simulink model "snap2_f_200msps_64i_4096c"  (R2019a)
settings: Solver=VariableStepDiscrete  StartTime=0.0  StopTime=10.0  RelTol=1e-3
undefined symbols (not defined in the file or in its folder): datetime, posixtime
libraries: xbsIndex_r4 x21354, casper_library_misc x297, casper_library_delays x19, xps_library x14, casper_library_sources x4
(part 151 of 217)

== system snap2_f_200msps_64i_4096c/cosmic_ray/buffer_and_packetizer/transpose/bus_create4 ==
  in1 : Inport
  in2 : Inport  Port=2
  concatenate : xbsIndex_r4/Concat  num_inputs=2  dbl_ovrd=off  block_type=concat
  reinterpret1 : xbsIndex_r4/Reinterpret  force_arith_type=on  arith_type=Unsigned  force_bin_pt=on  bin_pt=0  block_type=reinterpret
      settings: infoedit="Changes signal type without altering the binary representation.   You can changed the signal between signed and unsigned, and relocate the binary point.<br><br>Hardware notes: In hardware this block costs nothing.<br><br>Example:  Suppose the input is 6 bits wide, signed, with 2 fractional bits, and the output is forced to unsigned with 0 fractional bits.  Then an input of -2.0 (1110.00 in binary 2's complement) becomes an output of 56 (111000 in binary)."
  reinterpret2 : xbsIndex_r4/Reinterpret  force_arith_type=on  arith_type=Unsigned  force_bin_pt=on  bin_pt=0  block_type=reinterpret
      settings: infoedit="Changes signal type without altering the binary representation.   You can changed the signal between signed and unsigned, and relocate the binary point.<br><br>Hardware notes: In hardware this block costs nothing.<br><br>Example:  Suppose the input is 6 bits wide, signed, with 2 fractional bits, and the output is forced to unsigned with 0 fractional bits.  Then an input of -2.0 (1110.00 in binary 2's complement) becomes an output of 56 (111000 in binary)."
  bus_out : Outport
  wires:
  concatenate/1 -> bus_out/1
  in1/1 -> reinterpret1/1
  reinterpret1/1 -> concatenate/1
  in2/1 -> reinterpret2/1
  reinterpret2/1 -> concatenate/2

== system snap2_f_200msps_64i_4096c/cosmic_ray/buffer_and_packetizer/transpose/bus_create5 ==
  in1 : Inport
  in2 : Inport  Port=2
  concatenate : xbsIndex_r4/Concat  num_inputs=2  dbl_ovrd=off  block_type=concat
  reinterpret1 : xbsIndex_r4/Reinterpret  force_arith_type=on  arith_type=Unsigned  force_bin_pt=on  bin_pt=0  block_type=reinterpret
      settings: infoedit="Changes signal type without altering the binary representation.   You can changed the signal between signed and unsigned, and relocate the binary point.<br><br>Hardware notes: In hardware this block costs nothing.<br><br>Example:  Suppose the input is 6 bits wide, signed, with 2 fractional bits, and the output is forced to unsigned with 0 fractional bits.  Then an input of -2.0 (1110.00 in binary 2's complement) becomes an output of 56 (111000 in binary)."
  reinterpret2 : xbsIndex_r4/Reinterpret  force_arith_type=on  arith_type=Unsigned  force_bin_pt=on  bin_pt=0  block_type=reinterpret
      settings: infoedit="Changes signal type without altering the binary representation.   You can changed the signal between signed and unsigned, and relocate the binary point.<br><br>Hardware notes: In hardware this block costs nothing.<br><br>Example:  Suppose the input is 6 bits wide, signed, with 2 fractional bits, and the output is forced to unsigned with 0 fractional bits.  Then an input of -2.0 (1110.00 in binary 2's complement) becomes an output of 56 (111000 in binary)."
  bus_out : Outport
  wires:
  reinterpret2/1 -> concatenate/2
  in2/1 -> reinterpret2/1
  reinterpret1/1 -> concatenate/1
  in1/1 -> reinterpret1/1
  concatenate/1 -> bus_out/1

== system snap2_f_200msps_64i_4096c/cosmic_ray/buffer_and_packetizer/transpose/bus_create6 ==
  in1 : Inport
  in2 : Inport  Port=2
  concatenate : xbsIndex_r4/Concat  num_inputs=2  dbl_ovrd=off  block_type=concat
  reinterpret1 : xbsIndex_r4/Reinterpret  force_arith_type=on  arith_type=Unsigned  force_bin_pt=on  bin_pt=0  block_type=reinterpret
      settings: infoedit="Changes signal type without altering the binary representation.   You can changed the signal between signed and unsigned, and relocate the binary point.<br><br>Hardware notes: In hardware this block costs nothing.<br><br>Example:  Suppose the input is 6 bits wide, signed, with 2 fractional bits, and the output is forced to unsigned with 0 fractional bits.  Then an input of -2.0 (1110.00 in binary 2's complement) becomes an output of 56 (111000 in binary)."
  reinterpret2 : xbsIndex_r4/Reinterpret  force_arith_type=on  arith_type=Unsigned  force_bin_pt=on  bin_pt=0  block_type=reinterpret
      settings: infoedit="Changes signal type without altering the binary representation.   You can changed the signal between signed and unsigned, and relocate the binary point.<br><br>Hardware notes: In hardware this block costs nothing.<br><br>Example:  Suppose the input is 6 bits wide, signed, with 2 fractional bits, and the output is forced to unsigned with 0 fractional bits.  Then an input of -2.0 (1110.00 in binary 2's complement) becomes an output of 56 (111000 in binary)."
  bus_out : Outport
  wires:
  reinterpret2/1 -> concatenate/2
  in2/1 -> reinterpret2/1
  reinterpret1/1 -> concatenate/1
  in1/1 -> reinterpret1/1
  concatenate/1 -> bus_out/1

== system snap2_f_200msps_64i_4096c/cosmic_ray/buffer_and_packetizer/transpose/bus_create7 ==
  in1 : Inport
  in2 : Inport  Port=2
  concatenate : xbsIndex_r4/Concat  num_inputs=2  dbl_ovrd=off  block_type=concat
  reinterpret1 : xbsIndex_r4/Reinterpret  force_arith_type=on  arith_type=Unsigned  force_bin_pt=on  bin_pt=0  block_type=reinterpret
      settings: infoedit="Changes signal type without altering the binary representation.   You can changed the signal between signed and unsigned, and relocate the binary point.<br><br>Hardware notes: In hardware this block costs nothing.<br><br>Example:  Suppose the input is 6 bits wide, signed, with 2 fractional bits, and the output is forced to unsigned with 0 fractional bits.  Then an input of -2.0 (1110.00 in binary 2's complement) becomes an output of 56 (111000 in binary)."
  reinterpret2 : xbsIndex_r4/Reinterpret  force_arith_type=on  arith_type=Unsigned  force_bin_pt=on  bin_pt=0  block_type=reinterpret
      settings: infoedit="Changes signal type without altering the binary representation.   You can changed the signal between signed and unsigned, and relocate the binary point.<br><br>Hardware notes: In hardware this block costs nothing.<br><br>Example:  Suppose the input is 6 bits wide, signed, with 2 fractional bits, and the output is forced to unsigned with 0 fractional bits.  Then an input of -2.0 (1110.00 in binary 2's complement) becomes an output of 56 (111000 in binary)."
  bus_out : Outport
  wires:
  concatenate/1 -> bus_out/1
  in1/1 -> reinterpret1/1
  reinterpret1/1 -> concatenate/1
  in2/1 -> reinterpret2/1
  reinterpret2/1 -> concatenate/2

== system snap2_f_200msps_64i_4096c/cosmic_ray/buffer_and_packetizer/transpose/bus_create8 ==
  in1 : Inport
  in2 : Inport  Port=2
  concatenate : xbsIndex_r4/Concat  num_inputs=2  dbl_ovrd=off  block_type=concat
  reinterpret1 : xbsIndex_r4/Reinterpret  force_arith_type=on  arith_type=Unsigned  force_bin_pt=on  bin_pt=0  block_type=reinterpret
      settings: infoedit="Changes signal type without altering the binary representation.   You can changed the signal between signed and unsigned, and relocate the binary point.<br><br>Hardware notes: In hardware this block costs nothing.<br><br>Example:  Suppose the input is 6 bits wide, signed, with 2 fractional bits, and the output is forced to unsigned with 0 fractional bits.  Then an input of -2.0 (1110.00 in binary 2's complement) becomes an output of 56 (111000 in binary)."
  reinterpret2 : xbsIndex_r4/Reinterpret  force_arith_type=on  arith_type=Unsigned  force_bin_pt=on  bin_pt=0  block_type=reinterpret
      settings: infoedit="Changes signal type without altering the binary representation.   You can changed the signal between signed and unsigned, and relocate the binary point.<br><br>Hardware notes: In hardware this block costs nothing.<br><br>Example:  Suppose the input is 6 bits wide, signed, with 2 fractional bits, and the output is forced to unsigned with 0 fractional bits.  Then an input of -2.0 (1110.00 in binary 2's complement) becomes an output of 56 (111000 in binary)."
  bus_out : Outport
  wires:
  reinterpret2/1 -> concatenate/2
  in2/1 -> reinterpret2/1
  reinterpret1/1 -> concatenate/1
  in1/1 -> reinterpret1/1
  concatenate/1 -> bus_out/1

== system snap2_f_200msps_64i_4096c/cosmic_ray/buffer_and_packetizer/transpose/bus_expand2 ==
  bus_in : Inport
  reinterpret{1..16} (16 alike) : xbsIndex_r4/Reinterpret  force_arith_type=on  arith_type="Signed  (2's comp)"  force_bin_pt=on  bin_pt=0  block_type=reinterpret
  slice1 : xbsIndex_r4/Slice  nbits=10  boolean_output=off  mode=Upper Bit Location + Width  bit1=-150  base1=MSB of Input  bit0=0  base0=LSB of Input  dbl_ovrd=off  block_type=slice
  slice10 : xbsIndex_r4/Slice  nbits=10  boolean_output=off  mode=Upper Bit Location + Width  bit1=-60  base1=MSB of Input  bit0=0  base0=LSB of Input  dbl_ovrd=off  block_type=slice
  slice11 : xbsIndex_r4/Slice  nbits=10  boolean_output=off  mode=Upper Bit Location + Width  bit1=-50  base1=MSB of Input  bit0=0  base0=LSB of Input  dbl_ovrd=off  block_type=slice
  slice12 : xbsIndex_r4/Slice  nbits=10  boolean_output=off  mode=Upper Bit Location + Width  bit1=-40  base1=MSB of Input  bit0=0  base0=LSB of Input  dbl_ovrd=off  block_type=slice
  slice13 : xbsIndex_r4/Slice  nbits=10  boolean_output=off  mode=Upper Bit Location + Width  bit1=-30  base1=MSB of Input  bit0=0  base0=LSB of Input  dbl_ovrd=off  block_type=slice
  slice14 : xbsIndex_r4/Slice  nbits=10  boolean_output=off  mode=Upper Bit Location + Width  bit1=-20  base1=MSB of Input  bit0=0  base0=LSB of Input  dbl_ovrd=off  block_type=slice
  slice15 : xbsIndex_r4/Slice  nbits=10  boolean_output=off  mode=Upper Bit Location + Width  bit1=-10  base1=MSB of Input  bit0=0  base0=LSB of Input  dbl_ovrd=off  block_type=slice
  slice16 : xbsIndex_r4/Slice  nbits=10  boolean_output=off  mode=Upper Bit Location + Width  bit1=0  base1=MSB of Input  bit0=0  base0=LSB of Input  dbl_ovrd=off  block_type=slice
  slice2 : xbsIndex_r4/Slice  nbits=10  boolean_output=off  mode=Upper Bit Location + Width  bit1=-140  base1=MSB of Input  bit0=0  base0=LSB of Input  dbl_ovrd=off  block_type=slice
  slice3 : xbsIndex_r4/Slice  nbits=10  boolean_output=off  mode=Upper Bit Location + Width  bit1=-130  base1=MSB of Input  bit0=0  base0=LSB of Input  dbl_ovrd=off  block_type=slice
  slice4 : xbsIndex_r4/Slice  nbits=10  boolean_output=off  mode=Upper Bit Location + Width  bit1=-120  base1=MSB of Input  bit0=0  base0=LSB of Input  dbl_ovrd=off  block_type=slice
  slice5 : xbsIndex_r4/Slice  nbits=10  boolean_output=off  mode=Upper Bit Location + Width  bit1=-110  base1=MSB of Input  bit0=0  base0=LSB of Input  dbl_ovrd=off  block_type=slice
  slice6 : xbsIndex_r4/Slice  nbits=10  boolean_output=off  mode=Upper Bit Location + Width  bit1=-100  base1=MSB of Input  bit0=0  base0=LSB of Input  dbl_ovrd=off  block_type=slice
  slice7 : xbsIndex_r4/Slice  nbits=10  boolean_output=off  mode=Upper Bit Location + Width  bit1=-90  base1=MSB of Input  bit0=0  base0=LSB of Input  dbl_ovrd=off  block_type=slice
  slice8 : xbsIndex_r4/Slice  nbits=10  boolean_output=off  mode=Upper Bit Location + Width  bit1=-80  base1=MSB of Input  bit0=0  base0=LSB of Input  dbl_ovrd=off  block_type=slice
  slice9 : xbsIndex_r4/Slice  nbits=10  boolean_output=off  mode=Upper Bit Location + Width  bit1=-70  base1=MSB of Input  bit0=0  base0=LSB of Input  dbl_ovrd=off  block_type=slice
  msb_out16 : Outport
  out15 : Outport  Port=2
  out14 : Outport  Port=3
  out13 : Outport  Port=4
  out12 : Outport  Port=5
  out11 : Outport  Port=6
  out10 : Outport  Port=7
  out9 : Outport  Port=8
  out8 : Outport  Port=9
  out7 : Outport  Port=10
  out6 : Outport  Port=11
  out5 : Outport  Port=12
  out4 : Outport  Port=13
  out3 : Outport  Port=14
  out2 : Outport  Port=15
  lsb_out1 : Outport  Port=16
  wires:
  bus_in/1 -> slice16/1, slice15/1, slice14/1, slice13/1, slice12/1, slice11/1, slice10/1, slice9/1, slice8/1, slice7/1, slice6/1, slice5/1, slice4/1, slice3/1, slice2/1, slice1/1
  slice16/1 -> reinterpret16/1
  reinterpret16/1 -> msb_out16/1
  slice15/1 -> reinterpret15/1
  reinterpret15/1 -> out15/1
  slice14/1 -> reinterpret14/1
  reinterpret14/1 -> out14/1
  slice13/1 -> reinterpret13/1
  reinterpret13/1 -> out13/1
  slice12/1 -> reinterpret12/1
  reinterpret12/1 -> out12/1
  slice11/1 -> reinterpret11/1
  reinterpret11/1 -> out11/1
  slice10/1 -> reinterpret10/1
  reinterpret10/1 -> out10/1
  slice9/1 -> reinterpret9/1
  reinterpret9/1 -> out9/1
  slice8/1 -> reinterpret8/1
  reinterpret8/1 -> out8/1
  slice7/1 -> reinterpret7/1
  reinterpret7/1 -> out7/1
  slice6/1 -> reinterpret6/1
  reinterpret6/1 -> out6/1
  slice5/1 -> reinterpret5/1
  reinterpret5/1 -> out5/1
  slice4/1 -> reinterpret4/1
  reinterpret4/1 -> out4/1
  slice3/1 -> reinterpret3/1
  reinterpret3/1 -> out3/1
  slice2/1 -> reinterpret2/1
  reinterpret2/1 -> out2/1
  slice1/1 -> reinterpret1/1
  reinterpret1/1 -> lsb_out1/1

== system snap2_f_200msps_64i_4096c/cosmic_ray/buffer_and_packetizer/transpose/square_transposer ==
  sync : Inport
  in0 : Inport  Port=2
  in1 : Inport  Port=3
  in2 : Inport  Port=4
  in3 : Inport  Port=5
  in4 : Inport  Port=6
  in5 : Inport  Port=7
  in6 : Inport  Port=8
  in7 : Inport  Port=9
  barrel_switcher : Subsystem  AncestorBlock=casper_library_reorder/barrel_switcher  mask(barrel_switcher){n_inputs=3, async=off}
      mask prompts: n_inputs "Number of Inputs: (2^?)"; async "Asynchronous operation"
      mask help:
      | Shifts input to right by amount specified on sel,
      | wrapping around into higher order bits.
      mask init:
      | barrel_switcher_init(gcb,...
      |     'n_inputs', n_inputs, ...
      |     'async', async);
      mask Help: eval('xlWeb(''http://casper.berkeley.edu/wiki/Barrel_switcher'')')
  counter : xbsIndex_r4/Counter  cnt_type=Free Running  cnt_to=Inf  operation=Down  start_count=0  cnt_by_val=1  arith_type=Unsigned  n_bits=n_inputs  bin_pt=0  load_pin=off  rst=on  en=off  explicit_period=on  period=1  use_behavioral_HDL=off  implementation=Fabric  dbl_ovrd=off  block_type=counter
  db0 : Subsystem  AncestorBlock=casper_library_delays/delay_slr  mask(delay_slr){DelayLen=7, async=off}
      mask prompts: DelayLen "Delay by:"; async "asynchronous operation"
      mask help: A delay block that uses slices (SLR16s) for its storage.
      mask init:
      | delay_slr_init(gcb, ...
      |     'DelayLen', DelayLen, ...
      |     'async', async);
  db1 : Subsystem  AncestorBlock=casper_library_delays/delay_slr  mask(delay_slr){DelayLen=6, async=off}
      mask prompts: DelayLen "Delay by:"; async "asynchronous operation"
      mask help: A delay block that uses slices (SLR16s) for its storage.
      mask init:
      | delay_slr_init(gcb, ...
      |     'DelayLen', DelayLen, ...
      |     'async', async);
  db2 : Subsystem  AncestorBlock=casper_library_delays/delay_slr  mask(delay_slr){DelayLen=5, async=off}
      mask prompts: DelayLen "Delay by:"; async "asynchronous operation"
      mask help: A delay block that uses slices (SLR16s) for its storage.
      mask init:
      | delay_slr_init(gcb, ...
      |     'DelayLen', DelayLen, ...
      |     'async', async);
  db3 : Subsystem  AncestorBlock=casper_library_delays/delay_slr  mask(delay_slr){DelayLen=4, async=off}
      mask prompts: DelayLen "Delay by:"; async "asynchronous operation"
      mask help: A delay block that uses slices (SLR16s) for its storage.
      mask init:
      | delay_slr_init(gcb, ...
      |     'DelayLen', DelayLen, ...
      |     'async', async);
  db4 : Subsystem  AncestorBlock=casper_library_delays/delay_slr  mask(delay_slr){DelayLen=3, async=off}
      mask prompts: DelayLen "Delay by:"; async "asynchronous operation"
      mask help: A delay block that uses slices (SLR16s) for its storage.
      mask init:
      | delay_slr_init(gcb, ...
      |     'DelayLen', DelayLen, ...
      |     'async', async);
  db5 : Subsystem  AncestorBlock=casper_library_delays/delay_slr  mask(delay_slr){DelayLen=2, async=off}
      mask prompts: DelayLen "Delay by:"; async "asynchronous operation"
      mask help: A delay block that uses slices (SLR16s) for its storage.
      mask init:
      | delay_slr_init(gcb, ...
      |     'DelayLen', DelayLen, ...
      |     'async', async);
  db6 : Subsystem  AncestorBlock=casper_library_delays/delay_slr  mask(delay_slr){DelayLen=1, async=off}
      mask prompts: DelayLen "Delay by:"; async "asynchronous operation"
      mask help: A delay block that uses slices (SLR16s) for its storage.
      mask init:
      | delay_slr_init(gcb, ...
      |     'DelayLen', DelayLen, ...
      |     'async', async);
  df1 : Subsystem  AncestorBlock=casper_library_delays/delay_slr  mask(delay_slr){DelayLen=1, async=off}
      mask prompts: DelayLen "Delay by:"; async "asynchronous operation"
      mask help: A delay block that uses slices (SLR16s) for its storage.
      mask init:
      | delay_slr_init(gcb, ...
      |     'DelayLen', DelayLen, ...
      |     'async', async);
  df2 : Subsystem  AncestorBlock=casper_library_delays/delay_slr  mask(delay_slr){DelayLen=2, async=off}
      mask prompts: DelayLen "Delay by:"; async "asynchronous operation"
      mask help: A delay block that uses slices (SLR16s) for its storage.
      mask init:
      | delay_slr_init(gcb, ...
      |     'DelayLen', DelayLen, ...
      |     'async', async);
  df3 : Subsystem  AncestorBlock=casper_library_delays/delay_slr  mask(delay_slr){DelayLen=3, async=off}
      mask prompts: DelayLen "Delay by:"; async "asynchronous operation"
      mask help: A delay block that uses slices (SLR16s) for its storage.
      mask init:
      | delay_slr_init(gcb, ...
      |     'DelayLen', DelayLen, ...
      |     'async', async);
  df4 : Subsystem  AncestorBlock=casper_library_delays/delay_slr  mask(delay_slr){DelayLen=4, async=off}
      mask prompts: DelayLen "Delay by:"; async "asynchronous operation"
      mask help: A delay block that uses slices (SLR16s) for its storage.
      mask init:
      | delay_slr_init(gcb, ...
      |     'DelayLen', DelayLen, ...
      |     'async', async);
  df5 : Subsystem  AncestorBlock=casper_library_delays/delay_slr  mask(delay_slr){DelayLen=5, async=off}
      mask prompts: DelayLen "Delay by:"; async "asynchronous operation"
      mask help: A delay block that uses slices (SLR16s) for its storage.
      mask init:
      | delay_slr_init(gcb, ...
      |     'DelayLen', DelayLen, ...
      |     'async', async);
  df6 : Subsystem  AncestorBlock=casper_library_delays/delay_slr  mask(delay_slr){DelayLen=6, async=off}
      mask prompts: DelayLen "Delay by:"; async "asynchronous operation"
      mask help: A delay block that uses slices (SLR16s) for its storage.
      mask init:
      | delay_slr_init(gcb, ...
      |     'DelayLen', DelayLen, ...
      |     'async', async);
  df7 : Subsystem  AncestorBlock=casper_library_delays/delay_slr  mask(delay_slr){DelayLen=7, async=off}
      mask prompts: DelayLen "Delay by:"; async "asynchronous operation"
      mask help: A delay block that uses slices (SLR16s) for its storage.
      mask init:
      | delay_slr_init(gcb, ...
      |     'DelayLen', DelayLen, ...
      |     'async', async);
  dsync : Subsystem  AncestorBlock=casper_library_delays/delay_slr  mask(delay_slr){DelayLen=7, async=off}
      mask prompts: DelayLen "Delay by:"; async "asynchronous operation"
      mask help: A delay block that uses slices (SLR16s) for its storage.
      mask init:
      | delay_slr_init(gcb, ...
      |     'DelayLen', DelayLen, ...
      |     'async', async);
  sync_out : Outport
  out0 : Outport  Port=2
  out1 : Outport  Port=3
  out2 : Outport  Port=4
  out3 : Outport  Port=5
  out4 : Outport  Port=6
  out5 : Outport  Port=7
  out6 : Outport  Port=8
  out7 : Outport  Port=9
  wires:
  sync/1 -> counter/1, barrel_switcher/2(sync_in)
  dsync/1(dout) -> sync_out/1
  counter/1 -> barrel_switcher/1(sel)
  barrel_switcher/1(sync_out) -> dsync/1(din)
  in0/1 -> barrel_switcher/3(In1)
  barrel_switcher/2(Out1) -> db0/1(din)
  db0/1(dout) -> out0/1
  in1/1 -> df1/1(din)
  df1/1(dout) -> barrel_switcher/10(In8)
  barrel_switcher/3(Out2) -> db1/1(din)
  db1/1(dout) -> out1/1
  in2/1 -> df2/1(din)
  df2/1(dout) -> barrel_switcher/9(In7)
  barrel_switcher/4(Out3) -> db2/1(din)
  db2/1(dout) -> out2/1
  in3/1 -> df3/1(din)
  df3/1(dout) -> barrel_switcher/8(In6)
  barrel_switcher/5(Out4) -> db3/1(din)
  db3/1(dout) -> out3/1
  in4/1 -> df4/1(din)
  df4/1(dout) -> barrel_switcher/7(In5)
  barrel_switcher/6(Out5) -> db4/1(din)
  db4/1(dout) -> out4/1
  in5/1 -> df5/1(din)
  df5/1(dout) -> barrel_switcher/6(In4)
  barrel_switcher/7(Out6) -> db5/1(din)
  db5/1(dout) -> out5/1
  in6/1 -> df6/1(din)
  df6/1(dout) -> barrel_switcher/5(In3)
  barrel_switcher/8(Out7) -> db6/1(din)
  db6/1(dout) -> out6/1
  in7/1 -> df7/1(din)
  df7/1(dout) -> barrel_switcher/4(In2)
  barrel_switcher/9(Out8) -> out7/1

== system snap2_f_200msps_64i_4096c/cosmic_ray/coincidence_trigger/4pt_avg/bus_addsub ==
  a : Inport
  b : Inport  Port=2
  a_debus : Subsystem  AncestorBlock=casper_library_flow_control/bus_expand  mask(bus_expand){mode=divisions of arbitrary size, outputNum=1, outputWidth=[24  24  24  24  24  24  24  24  24  24  24  24  24  24  24  24  24  24  24  24  24  24  24  24  24  24  24  24  24  24  24  24  24  24  24  24  24  24  24  24  24  24  24  24  24  24  24  24  24  24  24  24  24  24  24  24  24  24  24  24  24  24  24  24], outputBinaryPt=[0  0  0  0  0  0  0  0  0  0  0  0  0  0  0  0  0  0  0  0  0  0  0  0  0  0  0  0  0  0  0  0  0  0  0  0  0  0  0  0  0  0  0  0  0  0  0  0  0  0  0  0  0  0  0  0  0  0  0  0  0  0  0  0], outputArithmeticType=[1  1  1  1  1  1  1  1  1  1  1  1  1  1  1  1  1  1  1  1  1  1  1  1  1  1  1  1  1  1  1  1  1  1  1  1  1  1  1  1  1  1  1  1  1  1  1  1  1  1  1  1  1  1  1  1  1  1  1  1  1  1  1  1], show_format=on, outputToWorkspace=off, variablePrefix=, outputToModelAsWell=on}
      mask prompts: outputNum "Number of outputs:"; outputWidth "Output width [msb ... lsb]:"; outputBinaryPt "Output binary point position [msb ... lsb]:"; outputArithmeticType "Output arithmetic type (ufix=0, fix=1, bool=2) [msb ... lsb]:"; show_format "Print format string?"; outputToWorkspace "Output to workspace?"; variablePrefix "Variable name prefix:"; outputToModelAsWell "Output to model as well?"
      mask help:
      | Expands a 'bus' made using a bus_create or Xilinx
      | concat block.
      | The input will be divided into the specified number
      | of outputs with the specified arithmetic types.
      | Divisions are made from most significant bit.
      mask init: same as snap2_f_200msps_64i_4096c/autocorr/bus_expand
      settings: AttributesFormatString=64 outputs: f24.0,f24.0,f24.0,f24.0,f24.0,f24.0,f24.0,f24.0,f24.0,f24.0,f24.0,f24.0,f24.0,f24.0,f24.0,f24.0,f24.0,f24.0,f24.0,f24.0,f24.0,f24.0,f24.0,f24.0,f24.0,f24.0,f24.0,f24.0,f24.0,f24.0,f24.0,f24.0,f24.0,f24.0,f24.0,f24.0,f24.0,f24.0,f24.0,f24.0,f24.0,f24.0,f24.0,f24.0,f24.0,f24.0,f24.0,f24.0,f24.0,f24.0,f24.0,f24.0,f24.0,f24.0,f24.0,f24.0,f24.0,f24.0,f24.0,f24.0,f24.0,f24.0,f24.0,f24.0,
      mask TypeOptions mode: divisions of equal size | divisions of arbitrary size
      mask Callback mode: bus_expand_callback();
      mask Callback outputWidth: bus_expand_callback();
      mask Callback outputToWorkspace: bus_expand_callback();
  addsub{1..64} (64 alike) : xbsIndex_r4/AddSub  mode=Addition  use_carryin=off  use_carryout=off  en=off  latency=1  precision=User Defined  arith_type="Signed  (2's comp)"  n_bits=25  bin_pt=0  quantization=Truncate  overflow=Wrap  use_behavioral_HDL=on  hw_selection=Fabric  pipelined=on  dbl_ovrd=off  block_type=addsub
  b_debus : Subsystem  AncestorBlock=casper_library_flow_control/bus_expand  mask(bus_expand){mode=divisions of arbitrary size, outputNum=1, outputWidth=[24  24  24  24  24  24  24  24  24  24  24  24  24  24  24  24  24  24  24  24  24  24  24  24  24  24  24  24  24  24  24  24  24  24  24  24  24  24  24  24  24  24  24  24  24  24  24  24  24  24  24  24  24  24  24  24  24  24  24  24  24  24  24  24], outputBinaryPt=[0  0  0  0  0  0  0  0  0  0  0  0  0  0  0  0  0  0  0  0  0  0  0  0  0  0  0  0  0  0  0  0  0  0  0  0  0  0  0  0  0  0  0  0  0  0  0  0  0  0  0  0  0  0  0  0  0  0  0  0  0  0  0  0], outputArithmeticType=[1  1  1  1  1  1  1  1  1  1  1  1  1  1  1  1  1  1  1  1  1  1  1  1  1  1  1  1  1  1  1  1  1  1  1  1  1  1  1  1  1  1  1  1  1  1  1  1  1  1  1  1  1  1  1  1  1  1  1  1  1  1  1  1], show_format=on, outputToWorkspace=off, variablePrefix=, outputToModelAsWell=on}
      mask prompts: outputNum "Number of outputs:"; outputWidth "Output width [msb ... lsb]:"; outputBinaryPt "Output binary point position [msb ... lsb]:"; outputArithmeticType "Output arithmetic type (ufix=0, fix=1, bool=2) [msb ... lsb]:"; show_format "Print format string?"; outputToWorkspace "Output to workspace?"; variablePrefix "Variable name prefix:"; outputToModelAsWell "Output to model as well?"
      mask help:
      | Expands a 'bus' made using a bus_create or Xilinx
      | concat block.
      | The input will be divided into the specified number
      | of outputs with the specified arithmetic types.
      | Divisions are made from most significant bit.
      mask init: same as snap2_f_200msps_64i_4096c/autocorr/bus_expand
      settings: AttributesFormatString=64 outputs: f24.0,f24.0,f24.0,f24.0,f24.0,f24.0,f24.0,f24.0,f24.0,f24.0,f24.0,f24.0,f24.0,f24.0,f24.0,f24.0,f24.0,f24.0,f24.0,f24.0,f24.0,f24.0,f24.0,f24.0,f24.0,f24.0,f24.0,f24.0,f24.0,f24.0,f24.0,f24.0,f24.0,f24.0,f24.0,f24.0,f24.0,f24.0,f24.0,f24.0,f24.0,f24.0,f24.0,f24.0,f24.0,f24.0,f24.0,f24.0,f24.0,f24.0,f24.0,f24.0,f24.0,f24.0,f24.0,f24.0,f24.0,f24.0,f24.0,f24.0,f24.0,f24.0,f24.0,f24.0,
      mask TypeOptions mode: divisions of equal size | divisions of arbitrary size
      mask Callback mode: bus_expand_callback();
      mask Callback outputWidth: bus_expand_callback();
      mask Callback outputToWorkspace: bus_expand_callback();
  op_bussify : Subsystem  AncestorBlock=casper_library_flow_control/bus_create  mask(bus_create){inputNum=64}
      mask prompts: inputNum "Number of inputs:"
      mask init:
      | bus_create_init(gcb,...
      |     'inputNum', inputNum);
  dout : Outport
  wires:
  a/1 -> a_debus/1(bus_in)
  b/1 -> b_debus/1(bus_in)
  a_debus/1(msb_out64) -> addsub1/1
  b_debus/1(msb_out64) -> addsub1/2
  a_debus/2(out63) -> addsub2/1
  b_debus/2(out63) -> addsub2/2
  a_debus/3(out62) -> addsub3/1
  b_debus/3(out62) -> addsub3/2
  a_debus/4(out61) -> addsub4/1
  b_debus/4(out61) -> addsub4/2
  a_debus/5(out60) -> addsub5/1
  b_debus/5(out60) -> addsub5/2
  a_debus/6(out59) -> addsub6/1
  b_debus/6(out59) -> addsub6/2
  a_debus/7(out58) -> addsub7/1
  b_debus/7(out58) -> addsub7/2
  a_debus/8(out57) -> addsub8/1
  b_debus/8(out57) -> addsub8/2
  a_debus/9(out56) -> addsub9/1
  b_debus/9(out56) -> addsub9/2
  a_debus/10(out55) -> addsub10/1
  b_debus/10(out55) -> addsub10/2
  a_debus/11(out54) -> addsub11/1
  b_debus/11(out54) -> addsub11/2
  a_debus/12(out53) -> addsub12/1
  b_debus/12(out53) -> addsub12/2
  a_debus/13(out52) -> addsub13/1
  b_debus/13(out52) -> addsub13/2
  a_debus/14(out51) -> addsub14/1
  b_debus/14(out51) -> addsub14/2
  a_debus/15(out50) -> addsub15/1
  b_debus/15(out50) -> addsub15/2
  a_debus/16(out49) -> addsub16/1
  b_debus/16(out49) -> addsub16/2
  a_debus/17(out48) -> addsub17/1
  b_debus/17(out48) -> addsub17/2
  a_debus/18(out47) -> addsub18/1
  b_debus/18(out47) -> addsub18/2
  a_debus/19(out46) -> addsub19/1
  b_debus/19(out46) -> addsub19/2
  a_debus/20(out45) -> addsub20/1
  b_debus/20(out45) -> addsub20/2
  a_debus/21(out44) -> addsub21/1
  b_debus/21(out44) -> addsub21/2
  a_debus/22(out43) -> addsub22/1
  b_debus/22(out43) -> addsub22/2
  a_debus/23(out42) -> addsub23/1
  b_debus/23(out42) -> addsub23/2
  a_debus/24(out41) -> addsub24/1
  b_debus/24(out41) -> addsub24/2
  a_debus/25(out40) -> addsub25/1
  b_debus/25(out40) -> addsub25/2
  a_debus/26(out39) -> addsub26/1
  b_debus/26(out39) -> addsub26/2
  a_debus/27(out38) -> addsub27/1
  b_debus/27(out38) -> addsub27/2
  a_debus/28(out37) -> addsub28/1
  b_debus/28(out37) -> addsub28/2
  a_debus/29(out36) -> addsub29/1
  b_debus/29(out36) -> addsub29/2
  a_debus/30(out35) -> addsub30/1
  b_debus/30(out35) -> addsub30/2
  a_debus/31(out34) -> addsub31/1
  b_debus/31(out34) -> addsub31/2
  a_debus/32(out33) -> addsub32/1
  b_debus/32(out33) -> addsub32/2
  a_debus/33(out32) -> addsub33/1
  b_debus/33(out32) -> addsub33/2
  a_debus/34(out31) -> addsub34/1
  b_debus/34(out31) -> addsub34/2
  a_debus/35(out30) -> addsub35/1
  b_debus/35(out30) -> addsub35/2
  a_debus/36(out29) -> addsub36/1
  b_debus/36(out29) -> addsub36/2
  a_debus/37(out28) -> addsub37/1
  b_debus/37(out28) -> addsub37/2
  a_debus/38(out27) -> addsub38/1
  b_debus/38(out27) -> addsub38/2
  a_debus/39(out26) -> addsub39/1
  b_debus/39(out26) -> addsub39/2
  a_debus/40(out25) -> addsub40/1
  b_debus/40(out25) -> addsub40/2
  a_debus/41(out24) -> addsub41/1
  b_debus/41(out24) -> addsub41/2
  a_debus/42(out23) -> addsub42/1
  b_debus/42(out23) -> addsub42/2
  a_debus/43(out22) -> addsub43/1
  b_debus/43(out22) -> addsub43/2
  a_debus/44(out21) -> addsub44/1
  b_debus/44(out21) -> addsub44/2
  a_debus/45(out20) -> addsub45/1
  b_debus/45(out20) -> addsub45/2
  a_debus/46(out19) -> addsub46/1
  b_debus/46(out19) -> addsub46/2
  a_debus/47(out18) -> addsub47/1
  b_debus/47(out18) -> addsub47/2
  a_debus/48(out17) -> addsub48/1
  b_debus/48(out17) -> addsub48/2
  a_debus/49(out16) -> addsub49/1
  b_debus/49(out16) -> addsub49/2
  a_debus/50(out15) -> addsub50/1
  b_debus/50(out15) -> addsub50/2
  a_debus/51(out14) -> addsub51/1
  b_debus/51(out14) -> addsub51/2
  a_debus/52(out13) -> addsub52/1
  b_debus/52(out13) -> addsub52/2
  a_debus/53(out12) -> addsub53/1
  b_debus/53(out12) -> addsub53/2
  a_debus/54(out11) -> addsub54/1
  b_debus/54(out11) -> addsub54/2
  a_debus/55(out10) -> addsub55/1
  b_debus/55(out10) -> addsub55/2
  a_debus/56(out9) -> addsub56/1
  b_debus/56(out9) -> addsub56/2
  a_debus/57(out8) -> addsub57/1
  b_debus/57(out8) -> addsub57/2
  a_debus/58(out7) -> addsub58/1
  b_debus/58(out7) -> addsub58/2
  a_debus/59(out6) -> addsub59/1
  b_debus/59(out6) -> addsub59/2
  a_debus/60(out5) -> addsub60/1
  b_debus/60(out5) -> addsub60/2
  a_debus/61(out4) -> addsub61/1
  b_debus/61(out4) -> addsub61/2
  a_debus/62(out3) -> addsub62/1
  b_debus/62(out3) -> addsub62/2
  a_debus/63(out2) -> addsub63/1
  b_debus/63(out2) -> addsub63/2
  a_debus/64(lsb_out1) -> addsub64/1
  b_debus/64(lsb_out1) -> addsub64/2
  addsub1/1 -> op_bussify/1(in1)
  addsub2/1 -> op_bussify/2(in2)
  addsub3/1 -> op_bussify/3(in3)
  addsub4/1 -> op_bussify/4(in4)
  addsub5/1 -> op_bussify/5(in5)
  addsub6/1 -> op_bussify/6(in6)
  addsub7/1 -> op_bussify/7(in7)
  addsub8/1 -> op_bussify/8(in8)
  addsub9/1 -> op_bussify/9(in9)
  addsub10/1 -> op_bussify/10(in10)
  addsub11/1 -> op_bussify/11(in11)
  addsub12/1 -> op_bussify/12(in12)
  addsub13/1 -> op_bussify/13(in13)
  addsub14/1 -> op_bussify/14(in14)
  addsub15/1 -> op_bussify/15(in15)
  addsub16/1 -> op_bussify/16(in16)
  addsub17/1 -> op_bussify/17(in17)
  addsub18/1 -> op_bussify/18(in18)
  addsub19/1 -> op_bussify/19(in19)
  addsub20/1 -> op_bussify/20(in20)
  addsub21/1 -> op_bussify/21(in21)
  addsub22/1 -> op_bussify/22(in22)
  addsub23/1 -> op_bussify/23(in23)
  addsub24/1 -> op_bussify/24(in24)
  addsub25/1 -> op_bussify/25(in25)
  addsub26/1 -> op_bussify/26(in26)
  addsub27/1 -> op_bussify/27(in27)
  addsub28/1 -> op_bussify/28(in28)
  addsub29/1 -> op_bussify/29(in29)
  addsub30/1 -> op_bussify/30(in30)
  addsub31/1 -> op_bussify/31(in31)
  addsub32/1 -> op_bussify/32(in32)
  addsub33/1 -> op_bussify/33(in33)
  addsub34/1 -> op_bussify/34(in34)
  addsub35/1 -> op_bussify/35(in35)
  addsub36/1 -> op_bussify/36(in36)
  addsub37/1 -> op_bussify/37(in37)
  addsub38/1 -> op_bussify/38(in38)
  addsub39/1 -> op_bussify/39(in39)
  addsub40/1 -> op_bussify/40(in40)
  addsub41/1 -> op_bussify/41(in41)
  addsub42/1 -> op_bussify/42(in42)
  addsub43/1 -> op_bussify/43(in43)
  addsub44/1 -> op_bussify/44(in44)
  addsub45/1 -> op_bussify/45(in45)
  addsub46/1 -> op_bussify/46(in46)
  addsub47/1 -> op_bussify/47(in47)
  addsub48/1 -> op_bussify/48(in48)
  addsub49/1 -> op_bussify/49(in49)
  addsub50/1 -> op_bussify/50(in50)
  addsub51/1 -> op_bussify/51(in51)
  addsub52/1 -> op_bussify/52(in52)
  addsub53/1 -> op_bussify/53(in53)
  addsub54/1 -> op_bussify/54(in54)
  addsub55/1 -> op_bussify/55(in55)
  addsub56/1 -> op_bussify/56(in56)
  addsub57/1 -> op_bussify/57(in57)
  addsub58/1 -> op_bussify/58(in58)
  addsub59/1 -> op_bussify/59(in59)
  addsub60/1 -> op_bussify/60(in60)
  addsub61/1 -> op_bussify/61(in61)
  addsub62/1 -> op_bussify/62(in62)
  addsub63/1 -> op_bussify/63(in63)
  addsub64/1 -> op_bussify/64(in64)
  op_bussify/1(bus_out) -> dout/1

== system snap2_f_200msps_64i_4096c/cosmic_ray/coincidence_trigger/4pt_avg/bus_addsub1 ==
  a : Inport
  b : Inport  Port=2
  a_debus : Subsystem  AncestorBlock=casper_library_flow_control/bus_expand  mask(bus_expand){mode=divisions of arbitrary size, outputNum=1, outputWidth=[24  24  24  24  24  24  24  24  24  24  24  24  24  24  24  24  24  24  24  24  24  24  24  24  24  24  24  24  24  24  24  24  24  24  24  24  24  24  24  24  24  24  24  24  24  24  24  24  24  24  24  24  24  24  24  24  24  24  24  24  24  24  24  24], outputBinaryPt=[0  0  0  0  0  0  0  0  0  0  0  0  0  0  0  0  0  0  0  0  0  0  0  0  0  0  0  0  0  0  0  0  0  0  0  0  0  0  0  0  0  0  0  0  0  0  0  0  0  0  0  0  0  0  0  0  0  0  0  0  0  0  0  0], outputArithmeticType=[1  1  1  1  1  1  1  1  1  1  1  1  1  1  1  1  1  1  1  1  1  1  1  1  1  1  1  1  1  1  1  1  1  1  1  1  1  1  1  1  1  1  1  1  1  1  1  1  1  1  1  1  1  1  1  1  1  1  1  1  1  1  1  1], show_format=on, outputToWorkspace=off, variablePrefix=, outputToModelAsWell=on}
      mask prompts: outputNum "Number of outputs:"; outputWidth "Output width [msb ... lsb]:"; outputBinaryPt "Output binary point position [msb ... lsb]:"; outputArithmeticType "Output arithmetic type (ufix=0, fix=1, bool=2) [msb ... lsb]:"; show_format "Print format string?"; outputToWorkspace "Output to workspace?"; variablePrefix "Variable name prefix:"; outputToModelAsWell "Output to model as well?"
      mask help:
      | Expands a 'bus' made using a bus_create or Xilinx
      | concat block.
      | The input will be divided into the specified number
      | of outputs with the specified arithmetic types.
      | Divisions are made from most significant bit.
      mask init: same as snap2_f_200msps_64i_4096c/autocorr/bus_expand
      settings: AttributesFormatString=64 outputs: f24.0,f24.0,f24.0,f24.0,f24.0,f24.0,f24.0,f24.0,f24.0,f24.0,f24.0,f24.0,f24.0,f24.0,f24.0,f24.0,f24.0,f24.0,f24.0,f24.0,f24.0,f24.0,f24.0,f24.0,f24.0,f24.0,f24.0,f24.0,f24.0,f24.0,f24.0,f24.0,f24.0,f24.0,f24.0,f24.0,f24.0,f24.0,f24.0,f24.0,f24.0,f24.0,f24.0,f24.0,f24.0,f24.0,f24.0,f24.0,f24.0,f24.0,f24.0,f24.0,f24.0,f24.0,f24.0,f24.0,f24.0,f24.0,f24.0,f24.0,f24.0,f24.0,f24.0,f24.0,
      mask TypeOptions mode: divisions of equal size | divisions of arbitrary size
      mask Callback mode: bus_expand_callback();
      mask Callback outputWidth: bus_expand_callback();
      mask Callback outputToWorkspace: bus_expand_callback();
  addsub{1..64} (64 alike) : xbsIndex_r4/AddSub  mode=Addition  use_carryin=off  use_carryout=off  en=off  latency=1  precision=User Defined  arith_type="Signed  (2's comp)"  n_bits=25  bin_pt=0  quantization=Truncate  overflow=Wrap  use_behavioral_HDL=on  hw_selection=Fabric  pipelined=on  dbl_ovrd=off  block_type=addsub
  b_debus : Subsystem  AncestorBlock=casper_library_flow_control/bus_expand  mask(bus_expand){mode=divisions of arbitrary size, outputNum=1, outputWidth=[24  24  24  24  24  24  24  24  24  24  24  24  24  24  24  24  24  24  24  24  24  24  24  24  24  24  24  24  24  24  24  24  24  24  24  24  24  24  24  24  24  24  24  24  24  24  24  24  24  24  24  24  24  24  24  24  24  24  24  24  24  24  24  24], outputBinaryPt=[0  0  0  0  0  0  0  0  0  0  0  0  0  0  0  0  0  0  0  0  0  0  0  0  0  0  0  0  0  0  0  0  0  0  0  0  0  0  0  0  0  0  0  0  0  0  0  0  0  0  0  0  0  0  0  0  0  0  0  0  0  0  0  0], outputArithmeticType=[1  1  1  1  1  1  1  1  1  1  1  1  1  1  1  1  1  1  1  1  1  1  1  1  1  1  1  1  1  1  1  1  1  1  1  1  1  1  1  1  1  1  1  1  1  1  1  1  1  1  1  1  1  1  1  1  1  1  1  1  1  1  1  1], show_format=on, outputToWorkspace=off, variablePrefix=, outputToModelAsWell=on}
      mask prompts: outputNum "Number of outputs:"; outputWidth "Output width [msb ... lsb]:"; outputBinaryPt "Output binary point position [msb ... lsb]:"; outputArithmeticType "Output arithmetic type (ufix=0, fix=1, bool=2) [msb ... lsb]:"; show_format "Print format string?"; outputToWorkspace "Output to workspace?"; variablePrefix "Variable name prefix:"; outputToModelAsWell "Output to model as well?"
      mask help:
      | Expands a 'bus' made using a bus_create or Xilinx
      | concat block.
      | The input will be divided into the specified number
      | of outputs with the specified arithmetic types.
      | Divisions are made from most significant bit.
      mask init: same as snap2_f_200msps_64i_4096c/autocorr/bus_expand
      settings: AttributesFormatString=64 outputs: f24.0,f24.0,f24.0,f24.0,f24.0,f24.0,f24.0,f24.0,f24.0,f24.0,f24.0,f24.0,f24.0,f24.0,f24.0,f24.0,f24.0,f24.0,f24.0,f24.0,f24.0,f24.0,f24.0,f24.0,f24.0,f24.0,f24.0,f24.0,f24.0,f24.0,f24.0,f24.0,f24.0,f24.0,f24.0,f24.0,f24.0,f24.0,f24.0,f24.0,f24.0,f24.0,f24.0,f24.0,f24.0,f24.0,f24.0,f24.0,f24.0,f24.0,f24.0,f24.0,f24.0,f24.0,f24.0,f24.0,f24.0,f24.0,f24.0,f24.0,f24.0,f24.0,f24.0,f24.0,
      mask TypeOptions mode: divisions of equal size | divisions of arbitrary size
      mask Callback mode: bus_expand_callback();
      mask Callback outputWidth: bus_expand_callback();
      mask Callback outputToWorkspace: bus_expand_callback();
  op_bussify : Subsystem  AncestorBlock=casper_library_flow_control/bus_create  mask(bus_create){inputNum=64}
      mask prompts: inputNum "Number of inputs:"
      mask init:
      | bus_create_init(gcb,...
      |     'inputNum', inputNum);
  dout : Outport
  wires:
  op_bussify/1(bus_out) -> dout/1
  addsub64/1 -> op_bussify/64(in64)
  addsub63/1 -> op_bussify/63(in63)
  addsub62/1 -> op_bussify/62(in62)
  addsub61/1 -> op_bussify/61(in61)
  addsub60/1 -> op_bussify/60(in60)
  addsub59/1 -> op_bussify/59(in59)
  addsub58/1 -> op_bussify/58(in58)
  addsub57/1 -> op_bussify/57(in57)
  addsub56/1 -> op_bussify/56(in56)
  addsub55/1 -> op_bussify/55(in55)
  addsub54/1 -> op_bussify/54(in54)
  addsub53/1 -> op_bussify/53(in53)
  addsub52/1 -> op_bussify/52(in52)
  addsub51/1 -> op_bussify/51(in51)
  addsub50/1 -> op_bussify/50(in50)
  addsub49/1 -> op_bussify/49(in49)
  addsub48/1 -> op_bussify/48(in48)
  addsub47/1 -> op_bussify/47(in47)
  addsub46/1 -> op_bussify/46(in46)
  addsub45/1 -> op_bussify/45(in45)
  addsub44/1 -> op_bussify/44(in44)
  addsub43/1 -> op_bussify/43(in43)
  addsub42/1 -> op_bussify/42(in42)
  addsub41/1 -> op_bussify/41(in41)
  addsub40/1 -> op_bussify/40(in40)
  addsub39/1 -> op_bussify/39(in39)
  addsub38/1 -> op_bussify/38(in38)
  addsub37/1 -> op_bussify/37(in37)
  addsub36/1 -> op_bussify/36(in36)
  addsub35/1 -> op_bussify/35(in35)
  addsub34/1 -> op_bussify/34(in34)
  addsub33/1 -> op_bussify/33(in33)
  addsub32/1 -> op_bussify/32(in32)
  addsub31/1 -> op_bussify/31(in31)
  addsub30/1 -> op_bussify/30(in30)
  addsub29/1 -> op_bussify/29(in29)
  addsub28/1 -> op_bussify/28(in28)
  addsub27/1 -> op_bussify/27(in27)
  addsub26/1 -> op_bussify/26(in26)
  addsub25/1 -> op_bussify/25(in25)
  addsub24/1 -> op_bussify/24(in24)
  addsub23/1 -> op_bussify/23(in23)
  addsub22/1 -> op_bussify/22(in22)
  addsub21/1 -> op_bussify/21(in21)
  addsub20/1 -> op_bussify/20(in20)
  addsub19/1 -> op_bussify/19(in19)
  addsub18/1 -> op_bussify/18(in18)
  addsub17/1 -> op_bussify/17(in17)
  addsub16/1 -> op_bussify/16(in16)
  addsub15/1 -> op_bussify/15(in15)
  addsub14/1 -> op_bussify/14(in14)
  addsub13/1 -> op_bussify/13(in13)
  addsub12/1 -> op_bussify/12(in12)
  addsub11/1 -> op_bussify/11(in11)
  addsub10/1 -> op_bussify/10(in10)
  addsub9/1 -> op_bussify/9(in9)
  addsub8/1 -> op_bussify/8(in8)
  addsub7/1 -> op_bussify/7(in7)
  addsub6/1 -> op_bussify/6(in6)
  addsub5/1 -> op_bussify/5(in5)
  addsub4/1 -> op_bussify/4(in4)
  addsub3/1 -> op_bussify/3(in3)
  addsub2/1 -> op_bussify/2(in2)
  addsub1/1 -> op_bussify/1(in1)
  b_debus/64(lsb_out1) -> addsub64/2
  a_debus/64(lsb_out1) -> addsub64/1
  b_debus/63(out2) -> addsub63/2
  a_debus/63(out2) -> addsub63/1
  b_debus/62(out3) -> addsub62/2
  a_debus/62(out3) -> addsub62/1
  b_debus/61(out4) -> addsub61/2
  a_debus/61(out4) -> addsub61/1
  b_debus/60(out5) -> addsub60/2
  a_debus/60(out5) -> addsub60/1
  b_debus/59(out6) -> addsub59/2
  a_debus/59(out6) -> addsub59/1
  b_debus/58(out7) -> addsub58/2
  a_debus/58(out7) -> addsub58/1
  b_debus/57(out8) -> addsub57/2
  a_debus/57(out8) -> addsub57/1
  b_debus/56(out9) -> addsub56/2
  a_debus/56(out9) -> addsub56/1
  b_debus/55(out10) -> addsub55/2
  a_debus/55(out10) -> addsub55/1
  b_debus/54(out11) -> addsub54/2
  a_debus/54(out11) -> addsub54/1
  b_debus/53(out12) -> addsub53/2
  a_debus/53(out12) -> addsub53/1
  b_debus/52(out13) -> addsub52/2
  a_debus/52(out13) -> addsub52/1
  b_debus/51(out14) -> addsub51/2
  a_debus/51(out14) -> addsub51/1
  b_debus/50(out15) -> addsub50/2
  a_debus/50(out15) -> addsub50/1
  b_debus/49(out16) -> addsub49/2
  a_debus/49(out16) -> addsub49/1
  b_debus/48(out17) -> addsub48/2
  a_debus/48(out17) -> addsub48/1
  b_debus/47(out18) -> addsub47/2
  a_debus/47(out18) -> addsub47/1
  b_debus/46(out19) -> addsub46/2
  a_debus/46(out19) -> addsub46/1
  b_debus/45(out20) -> addsub45/2
  a_debus/45(out20) -> addsub45/1
  b_debus/44(out21) -> addsub44/2
  a_debus/44(out21) -> addsub44/1
  b_debus/43(out22) -> addsub43/2
  a_debus/43(out22) -> addsub43/1
  b_debus/42(out23) -> addsub42/2
  a_debus/42(out23) -> addsub42/1
  b_debus/41(out24) -> addsub41/2
  a_debus/41(out24) -> addsub41/1
  b_debus/40(out25) -> addsub40/2
  a_debus/40(out25) -> addsub40/1
  b_debus/39(out26) -> addsub39/2
  a_debus/39(out26) -> addsub39/1
  b_debus/38(out27) -> addsub38/2
  a_debus/38(out27) -> addsub38/1
  b_debus/37(out28) -> addsub37/2
  a_debus/37(out28) -> addsub37/1
  b_debus/36(out29) -> addsub36/2
  a_debus/36(out29) -> addsub36/1
  b_debus/35(out30) -> addsub35/2
  a_debus/35(out30) -> addsub35/1
  b_debus/34(out31) -> addsub34/2
  a_debus/34(out31) -> addsub34/1
  b_debus/33(out32) -> addsub33/2
  a_debus/33(out32) -> addsub33/1
  b_debus/32(out33) -> addsub32/2
  a_debus/32(out33) -> addsub32/1
  b_debus/31(out34) -> addsub31/2
  a_debus/31(out34) -> addsub31/1
  b_debus/30(out35) -> addsub30/2
  a_debus/30(out35) -> addsub30/1
  b_debus/29(out36) -> addsub29/2
  a_debus/29(out36) -> addsub29/1
  b_debus/28(out37) -> addsub28/2
  a_debus/28(out37) -> addsub28/1
  b_debus/27(out38) -> addsub27/2
  a_debus/27(out38) -> addsub27/1
  b_debus/26(out39) -> addsub26/2
  a_debus/26(out39) -> addsub26/1
  b_debus/25(out40) -> addsub25/2
  a_debus/25(out40) -> addsub25/1
  b_debus/24(out41) -> addsub24/2
  a_debus/24(out41) -> addsub24/1
  b_debus/23(out42) -> addsub23/2
  a_debus/23(out42) -> addsub23/1
  b_debus/22(out43) -> addsub22/2
  a_debus/22(out43) -> addsub22/1
  b_debus/21(out44) -> addsub21/2
  a_debus/21(out44) -> addsub21/1
  b_debus/20(out45) -> addsub20/2
  a_debus/20(out45) -> addsub20/1
  b_debus/19(out46) -> addsub19/2
  a_debus/19(out46) -> addsub19/1
  b_debus/18(out47) -> addsub18/2
  a_debus/18(out47) -> addsub18/1
  b_debus/17(out48) -> addsub17/2
  a_debus/17(out48) -> addsub17/1
  b_debus/16(out49) -> addsub16/2
  a_debus/16(out49) -> addsub16/1
  b_debus/15(out50) -> addsub15/2
  a_debus/15(out50) -> addsub15/1
  b_debus/14(out51) -> addsub14/2
  a_debus/14(out51) -> addsub14/1
  b_debus/13(out52) -> addsub13/2
  a_debus/13(out52) -> addsub13/1
  b_debus/12(out53) -> addsub12/2
  a_debus/12(out53) -> addsub12/1
  b_debus/11(out54) -> addsub11/2
  a_debus/11(out54) -> addsub11/1
  b_debus/10(out55) -> addsub10/2
  a_debus/10(out55) -> addsub10/1
  b_debus/9(out56) -> addsub9/2
  a_debus/9(out56) -> addsub9/1
  b_debus/8(out57) -> addsub8/2
  a_debus/8(out57) -> addsub8/1
  b_debus/7(out58) -> addsub7/2
  a_debus/7(out58) -> addsub7/1
  b_debus/6(out59) -> addsub6/2
  a_debus/6(out59) -> addsub6/1
  b_debus/5(out60) -> addsub5/2
  a_debus/5(out60) -> addsub5/1
  b_debus/4(out61) -> addsub4/2
  a_debus/4(out61) -> addsub4/1
  b_debus/3(out62) -> addsub3/2
  a_debus/3(out62) -> addsub3/1
  b_debus/2(out63) -> addsub2/2
  a_debus/2(out63) -> addsub2/1
  b_debus/1(msb_out64) -> addsub1/2
  a_debus/1(msb_out64) -> addsub1/1
  b/1 -> b_debus/1(bus_in)
  a/1 -> a_debus/1(bus_in)
